simulink model "Testailu_1stOderDelay"  (R2016b)
settings: Solver=FixedStepAuto  StartTime=0.0  StopTime=max(timeVector)  FixedStep=0.5  RelTol=1e-3
values from neighbouring files (symbols this model uses):
  t_delay_init = 1500    [dsa.m]
  Tau = 3700    [dsa.m]
  TotRange = abs(Values2 - Values1)    [dsa.m]
settings Model: Creator=maki9  LastModifiedBy=maki9

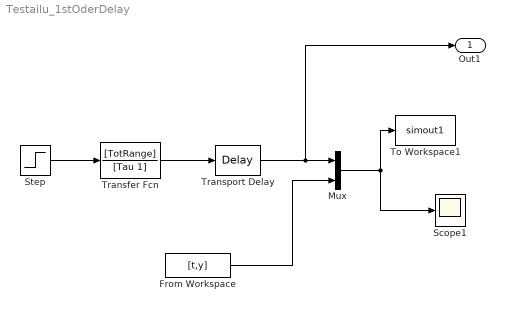
== system Testailu_1stOderDelay ==
  From Workspace : FromWorkspace  VariableName=[t,y]  SampleTime=0
  Mux : Mux  Inputs=2
  Scope1 : Scope
  Step : Step  SampleTime=0
  To Workspace1 : ToWorkspace  VariableName=simout1  SaveFormat=Timeseries  SampleTime=-1
  Transfer Fcn : TransferFcn  Numerator=[TotRange]  Denominator=[Tau 1]
  Transport Delay : TransportDelay  DelayTime=t_delay_init
  Out1 : Outport
  wires:
  Step/1 -> Transfer Fcn/1
  Transfer Fcn/1 -> Transport Delay/1
  Mux/1 -> Scope1/1, To Workspace1/1
  From Workspace/1 -> Mux/2
  Transport Delay/1 -> Out1/1, Mux/1
